simulink model "controller_sim"  (R2022a)
settings: Solver=ode1  StartTime=0.0  StopTime=10.0  FixedStep=0.010  RelTol=1e-5  AbsTol=1e-5
undefined symbols (not defined in the file or in its folder): c_d, c_dn, c_downbound, c_i, c_n, c_p, c_upbound, T0, T1, Td, Tg, Ti, Ts, Tsp, Tsp_delay, Tt
libraries: slpidlib x1
(part 2 of 3)

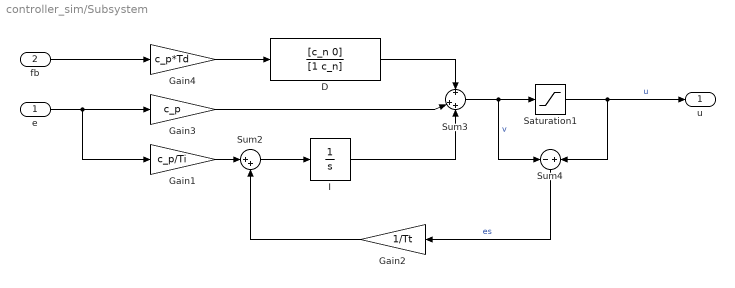
== system controller_sim/Subsystem ==
  e : Inport
  fb : Inport  Port=2
  D : TransferFcn  Numerator=[c_n 0]  Denominator=[1 c_n]
  Gain1 : Gain  Gain=c_p/Ti
  Gain2 : Gain  Gain=1/Tt
  Gain3 : Gain  Gain=c_p
  Gain4 : Gain  Gain=c_p*Td
  I : TransferFcn  Denominator=[1 0]
  Saturation1 : Saturate  UpperLimit=c_upbound  LowerLimit=c_downbound
  Sum2 : Sum  Inputs=|++
  Sum3 : Sum  Inputs=+|++
  Sum4 : Sum  Inputs=-|+
  u : Outport
  wires:
  D/1 -> Sum3/1
  e/1 -> Gain1/1, Gain3/1
  Sum2/1 -> I/1
  Gain4/1 -> D/1
  I/1 -> Sum3/3
  Gain3/1 -> Sum3/2
  Gain1/1 -> Sum2/1
  Saturation1/1 -> u/1, Sum4/2  "u"
  fb/1 -> Gain4/1
  Sum3/1 -> Sum4/1, Saturation1/1  "v"
  Gain2/1 -> Sum2/2
  Sum4/1 -> Gain2/1  "es"

== system controller_sim/Subsystem1 ==
  e : Inport
  fb : Inport  Port=2
  D : TransferFcn  Numerator=[c_n 0]  Denominator=[1 c_n]
  Gain1 : Gain  Gain=c_p/Ti
  Gain2 : Gain  Gain=1/Tt
  Gain3 : Gain  Gain=c_p
  Gain4 : Gain  Gain=c_p*Td
  I : TransferFcn  Denominator=[1 0]
  Saturation1 : Saturate  UpperLimit=c_upbound  LowerLimit=c_downbound
  Sum2 : Sum  Inputs=|++
  Sum3 : Sum  Inputs=+|++
  Sum4 : Sum  Inputs=-|+
  u : Outport
  wires:
  D/1 -> Sum3/1
  e/1 -> Gain1/1, Gain3/1
  Sum2/1 -> I/1
  Gain4/1 -> D/1
  I/1 -> Sum3/3
  Gain3/1 -> Sum3/2
  Gain1/1 -> Sum2/1
  Saturation1/1 -> u/1, Sum4/2  "u"
  fb/1 -> Gain4/1
  Sum3/1 -> Sum4/1, Saturation1/1  "v"
  Gain2/1 -> Sum2/2
  Sum4/1 -> Gain2/1  "es"

== system controller_sim/Subsystem10 ==
  e : Inport
  fb : Inport  Port=2
  D : TransferFcn  Numerator=[c_n]  Denominator=[1 c_n]
  Gain1 : Gain  Gain=c_p/Ti
  Gain2 : Gain  Gain=1/Tt
  Gain3 : Gain  Gain=c_p
  Gain4 : Gain  Gain=c_p*Td
  I : TransferFcn  Denominator=[1 0]
  Saturation1 : Saturate  UpperLimit=c_upbound  LowerLimit=c_downbound
  Sum2 : Sum  Inputs=|++
  Sum3 : Sum  Inputs=+|++
  Sum4 : Sum  Inputs=-|+
  u : Outport
  wires:
  D/1 -> Sum3/1
  e/1 -> Gain1/1, Gain3/1
  Sum2/1 -> I/1
  Gain4/1 -> D/1
  I/1 -> Sum3/3
  Gain3/1 -> Sum3/2
  Gain1/1 -> Sum2/1
  Saturation1/1 -> u/1, Sum4/2  "u"
  fb/1 -> Gain4/1
  Sum3/1 -> Sum4/1, Saturation1/1  "v"
  Gain2/1 -> Sum2/2
  Sum4/1 -> Gain2/1  "es"

== system controller_sim/Subsystem11 ==
  e : Inport
  fb : Inport  Port=2
  D : TransferFcn  Numerator=[c_n]  Denominator=[1 c_n]
  Gain1 : Gain  Gain=c_p/Ti
  Gain2 : Gain  Gain=1/Tt
  Gain3 : Gain  Gain=c_p
  Gain4 : Gain  Gain=c_p*Td
  I : TransferFcn  Denominator=[1 0]
  Saturation1 : Saturate  UpperLimit=c_upbound  LowerLimit=c_downbound
  Sum2 : Sum  Inputs=|++
  Sum3 : Sum  Inputs=+|++
  Sum4 : Sum  Inputs=-|+
  u : Outport
  wires:
  D/1 -> Sum3/1
  e/1 -> Gain1/1, Gain3/1
  Sum2/1 -> I/1
  Gain4/1 -> D/1
  I/1 -> Sum3/3
  Gain3/1 -> Sum3/2
  Gain1/1 -> Sum2/1
  Saturation1/1 -> u/1, Sum4/2  "u"
  fb/1 -> Gain4/1
  Sum3/1 -> Sum4/1, Saturation1/1  "v"
  Gain2/1 -> Sum2/2
  Sum4/1 -> Gain2/1  "es"

== system controller_sim/Subsystem12 ==
  e : Inport
  fb : Inport  Port=2
  D : TransferFcn  Numerator=[c_n]  Denominator=[1 c_n]
  Gain1 : Gain  Gain=c_p/Ti
  Gain2 : Gain  Gain=1/Tt
  Gain3 : Gain  Gain=c_p
  Gain4 : Gain  Gain=c_p*Td
  I : TransferFcn  Denominator=[1 0]
  Saturation1 : Saturate  UpperLimit=c_upbound  LowerLimit=c_downbound
  Sum2 : Sum  Inputs=|++
  Sum3 : Sum  Inputs=+|++
  Sum4 : Sum  Inputs=-|+
  u : Outport
  wires:
  D/1 -> Sum3/1
  e/1 -> Gain1/1, Gain3/1
  Sum2/1 -> I/1
  Gain4/1 -> D/1
  I/1 -> Sum3/3
  Gain3/1 -> Sum3/2
  Gain1/1 -> Sum2/1
  Saturation1/1 -> u/1, Sum4/2  "u"
  fb/1 -> Gain4/1
  Sum3/1 -> Sum4/1, Saturation1/1  "v"
  Gain2/1 -> Sum2/2
  Sum4/1 -> Gain2/1  "es"

== system controller_sim/Subsystem13 ==
  e : Inport
  fb : Inport  Port=2
  D : TransferFcn  Numerator=[c_n 0]  Denominator=[1 c_n]
  Gain1 : Gain  Gain=c_p/Ti
  Gain2 : Gain  Gain=1/Tt
  Gain3 : Gain  Gain=c_p
  Gain4 : Gain  Gain=c_p*Td
  I : TransferFcn  Denominator=[1 0]
  Saturation1 : Saturate  UpperLimit=c_upbound  LowerLimit=c_downbound
  Sum2 : Sum  Inputs=|++
  Sum3 : Sum  Inputs=+|++
  Sum4 : Sum  Inputs=-|+
  u : Outport
  wires:
  D/1 -> Sum3/1
  Sum2/1 -> I/1
  Gain4/1 -> D/1
  I/1 -> Sum3/3
  Gain3/1 -> Sum3/2
  Gain1/1 -> Sum2/1
  Saturation1/1 -> u/1, Sum4/2  "u"
  e/1 -> Gain4/1, Gain1/1, Gain3/1
  Sum3/1 -> Sum4/1, Saturation1/1  "v"
  Gain2/1 -> Sum2/2
  Sum4/1 -> Gain2/1  "es"

== system controller_sim/Subsystem14 ==
  e : Inport
  fb : Inport  Port=2
  D : TransferFcn  Numerator=[c_n 0]  Denominator=[1 c_n]
  Gain1 : Gain  Gain=c_p/Ti
  Gain2 : Gain  Gain=1/Tt
  Gain3 : Gain  Gain=c_p
  Gain4 : Gain  Gain=c_p*Td
  I : TransferFcn  Denominator=[1 0]
  Saturation1 : Saturate  UpperLimit=c_upbound  LowerLimit=c_downbound
  Sum2 : Sum  Inputs=|++
  Sum3 : Sum  Inputs=+|++
  Sum4 : Sum  Inputs=-|+
  u : Outport
  wires:
  D/1 -> Sum3/1
  Sum2/1 -> I/1
  Gain4/1 -> D/1
  I/1 -> Sum3/3
  Gain3/1 -> Sum3/2
  Gain1/1 -> Sum2/1
  Saturation1/1 -> u/1, Sum4/2  "u"
  e/1 -> Gain4/1, Gain1/1, Gain3/1
  Sum3/1 -> Sum4/1, Saturation1/1  "v"
  Gain2/1 -> Sum2/2
  Sum4/1 -> Gain2/1  "es"

== system controller_sim/Subsystem15 ==
  e : Inport
  fb : Inport  Port=2
  D : TransferFcn  Numerator=[c_n 0]  Denominator=[1 c_n]
  Gain1 : Gain  Gain=c_p/Ti
  Gain2 : Gain  Gain=1/Tt
  Gain3 : Gain  Gain=c_p
  Gain4 : Gain  Gain=c_p*Td
  I : TransferFcn  Denominator=[1 0]
  Saturation1 : Saturate  UpperLimit=c_upbound  LowerLimit=c_downbound
  Sum2 : Sum  Inputs=|++
  Sum3 : Sum  Inputs=+|++
  Sum4 : Sum  Inputs=-|+
  u : Outport
  wires:
  Sum4/1 -> Gain2/1  "es"
  Gain2/1 -> Sum2/2
  Sum3/1 -> Saturation1/1, Sum4/1  "v"
  e/1 -> Gain3/1, Gain1/1, Gain4/1
  Saturation1/1 -> Sum4/2, u/1  "u"
  Gain1/1 -> Sum2/1
  Gain3/1 -> Sum3/2
  I/1 -> Sum3/3
  Gain4/1 -> D/1
  Sum2/1 -> I/1
  D/1 -> Sum3/1

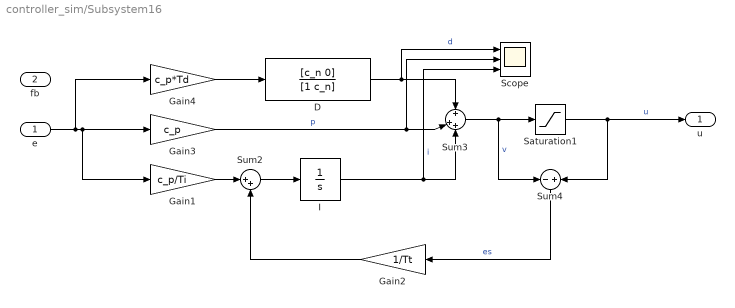
== system controller_sim/Subsystem16 ==
  e : Inport
  fb : Inport  Port=2
  D : TransferFcn  Numerator=[c_n 0]  Denominator=[1 c_n]
  Gain1 : Gain  Gain=c_p/Ti
  Gain2 : Gain  Gain=1/Tt
  Gain3 : Gain  Gain=c_p
  Gain4 : Gain  Gain=c_p*Td
  I : TransferFcn  Denominator=[1 0]
  Saturation1 : Saturate  UpperLimit=c_upbound  LowerLimit=c_downbound
  Scope : Scope  NumInputPorts=3
  Sum2 : Sum  Inputs=|++
  Sum3 : Sum  Inputs=+|++
  Sum4 : Sum  Inputs=-|+
  u : Outport
  wires:
  D/1 -> Scope/1, Sum3/1  "d"
  Sum2/1 -> I/1
  Gain4/1 -> D/1
  I/1 -> Scope/3, Sum3/3  "i"
  Gain3/1 -> Scope/2, Sum3/2  "p"
  Gain1/1 -> Sum2/1
  Saturation1/1 -> u/1, Sum4/2  "u"
  e/1 -> Gain4/1, Gain1/1, Gain3/1
  Sum3/1 -> Sum4/1, Saturation1/1  "v"
  Gain2/1 -> Sum2/2
  Sum4/1 -> Gain2/1  "es"

== system controller_sim/Subsystem17 ==
  e : Inport
  fb : Inport  Port=2
  D : TransferFcn  Numerator=[c_n 0]  Denominator=[1 c_n]
  Gain1 : Gain  Gain=c_p/Ti
  Gain2 : Gain  Gain=1/Tt
  Gain3 : Gain  Gain=c_p
  Gain4 : Gain  Gain=c_p*Td
  I : TransferFcn  Denominator=[1 0]
  Saturation1 : Saturate  UpperLimit=c_upbound  LowerLimit=c_downbound
  Sum2 : Sum  Inputs=|++
  Sum3 : Sum  Inputs=+|++
  Sum4 : Sum  Inputs=-|+
  u : Outport
  wires:
  Sum4/1 -> Gain2/1  "es"
  Gain2/1 -> Sum2/2
  Sum3/1 -> Saturation1/1, Sum4/1  "v"
  e/1 -> Gain3/1, Gain1/1, Gain4/1
  Saturation1/1 -> Sum4/2, u/1  "u"
  Gain1/1 -> Sum2/1
  Gain3/1 -> Sum3/2
  I/1 -> Sum3/3
  Gain4/1 -> D/1
  Sum2/1 -> I/1
  D/1 -> Sum3/1

== system controller_sim/Subsystem18 ==
  e : Inport
  fb : Inport  Port=2
  D : TransferFcn  Numerator=[c_n 0]  Denominator=[1 c_n]
  Gain1 : Gain  Gain=c_p/Ti
  Gain2 : Gain  Gain=1/Tt
  Gain3 : Gain  Gain=c_p
  Gain4 : Gain  Gain=c_p*Td
  I : TransferFcn  Denominator=[1 0]
  Saturation1 : Saturate  UpperLimit=c_upbound  LowerLimit=c_downbound
  Sum2 : Sum  Inputs=|++
  Sum3 : Sum  Inputs=+|++
  Sum4 : Sum  Inputs=-|+
  u : Outport
  wires:
  D/1 -> Sum3/1
  Sum2/1 -> I/1
  Gain4/1 -> D/1
  I/1 -> Sum3/3
  Gain3/1 -> Sum3/2
  Gain1/1 -> Sum2/1
  Saturation1/1 -> u/1, Sum4/2  "u"
  e/1 -> Gain4/1, Gain1/1, Gain3/1
  Sum3/1 -> Sum4/1, Saturation1/1  "v"
  Gain2/1 -> Sum2/2
  Sum4/1 -> Gain2/1  "es"

== system controller_sim/Subsystem19 ==
  e : Inport
  fb : Inport  Port=2
  D : TransferFcn  Numerator=[c_n 0]  Denominator=[1 c_n]
  Gain1 : Gain  Gain=c_p/Ti
  Gain2 : Gain  Gain=1/Tt
  Gain3 : Gain  Gain=c_p
  Gain4 : Gain  Gain=c_p*Td
  I : TransferFcn  Denominator=[1 0]
  Saturation1 : Saturate  UpperLimit=c_upbound  LowerLimit=c_downbound
  Sum2 : Sum  Inputs=|++
  Sum3 : Sum  Inputs=+|++
  Sum4 : Sum  Inputs=-|+
  u : Outport
  wires:
  Sum4/1 -> Gain2/1  "es"
  Gain2/1 -> Sum2/2
  Sum3/1 -> Saturation1/1, Sum4/1  "v"
  e/1 -> Gain3/1, Gain1/1, Gain4/1
  Saturation1/1 -> Sum4/2, u/1  "u"
  Gain1/1 -> Sum2/1
  Gain3/1 -> Sum3/2
  I/1 -> Sum3/3
  Gain4/1 -> D/1
  Sum2/1 -> I/1
  D/1 -> Sum3/1

== system controller_sim/Subsystem2 ==
  e : Inport
  fb : Inport  Port=2
  D : TransferFcn  Numerator=[c_n 0]  Denominator=[1 c_n]
  Gain1 : Gain  Gain=c_p/Ti
  Gain2 : Gain  Gain=1/Tt
  Gain3 : Gain  Gain=c_p
  Gain4 : Gain  Gain=c_p*Td
  I : TransferFcn  Denominator=[1 0]
  Saturation1 : Saturate  UpperLimit=c_upbound  LowerLimit=c_downbound
  Sum2 : Sum  Inputs=|++
  Sum3 : Sum  Inputs=+|++
  Sum4 : Sum  Inputs=-|+
  u : Outport
  wires:
  Sum4/1 -> Gain2/1  "es"
  Gain2/1 -> Sum2/2
  Sum3/1 -> Saturation1/1, Sum4/1  "v"
  fb/1 -> Gain4/1
  Saturation1/1 -> Sum4/2, u/1  "u"
  Gain1/1 -> Sum2/1
  Gain3/1 -> Sum3/2
  I/1 -> Sum3/3
  Gain4/1 -> D/1
  Sum2/1 -> I/1
  e/1 -> Gain3/1, Gain1/1
  D/1 -> Sum3/1

== system controller_sim/Subsystem22 ==
  e : Inport
  fb : Inport  Port=2
  D : TransferFcn  Numerator=[c_n 0]  Denominator=[1 c_n]
  Gain1 : Gain  Gain=c_p/Ti
  Gain2 : Gain  Gain=1/Tt
  Gain3 : Gain  Gain=c_p
  Gain4 : Gain  Gain=c_p*Td
  I : TransferFcn  Denominator=[1 0]
  Saturation1 : Saturate  UpperLimit=c_upbound  LowerLimit=c_downbound
  Sum2 : Sum  Inputs=|++
  Sum3 : Sum  Inputs=+|++
  Sum4 : Sum  Inputs=-|+
  u : Outport
  wires:
  Sum4/1 -> Gain2/1  "es"
  Gain2/1 -> Sum2/2
  Sum3/1 -> Saturation1/1, Sum4/1  "v"
  e/1 -> Gain3/1, Gain1/1, Gain4/1
  Saturation1/1 -> Sum4/2, u/1  "u"
  Gain1/1 -> Sum2/1
  Gain3/1 -> Sum3/2
  I/1 -> Sum3/3
  Gain4/1 -> D/1
  Sum2/1 -> I/1
  D/1 -> Sum3/1

== system controller_sim/Subsystem3 ==
  e : Inport
  fb : Inport  Port=2
  D : TransferFcn  Numerator=[c_n 0]  Denominator=[1 c_n]
  Gain1 : Gain  Gain=c_p/Ti
  Gain2 : Gain  Gain=1/Tt
  Gain3 : Gain  Gain=c_p
  Gain4 : Gain  Gain=c_p*Td
  I : TransferFcn  Denominator=[1 0]
  Saturation1 : Saturate  UpperLimit=c_upbound  LowerLimit=c_downbound
  Sum2 : Sum  Inputs=|++
  Sum3 : Sum  Inputs=+|++
  Sum4 : Sum  Inputs=-|+
  u : Outport
  wires:
  D/1 -> Sum3/1
  e/1 -> Gain1/1, Gain3/1
  Sum2/1 -> I/1
  Gain4/1 -> D/1
  I/1 -> Sum3/3
  Gain3/1 -> Sum3/2
  Gain1/1 -> Sum2/1
  Saturation1/1 -> u/1, Sum4/2  "u"
  fb/1 -> Gain4/1
  Sum3/1 -> Sum4/1, Saturation1/1  "v"
  Gain2/1 -> Sum2/2
  Sum4/1 -> Gain2/1  "es"

== system controller_sim/Subsystem4 ==
  e : Inport
  fb : Inport  Port=2
  D : TransferFcn  Numerator=[c_n]  Denominator=[1 c_n]
  Gain1 : Gain  Gain=c_p/Ti
  Gain2 : Gain  Gain=1/Tt
  Gain3 : Gain  Gain=c_p
  Gain4 : Gain  Gain=c_p*Td
  I : TransferFcn  Denominator=[1 0]
  Saturation1 : Saturate  UpperLimit=c_upbound  LowerLimit=c_downbound
  Sum2 : Sum  Inputs=|++
  Sum3 : Sum  Inputs=+|++
  Sum4 : Sum  Inputs=-|+
  u : Outport
  wires:
  D/1 -> Sum3/1
  e/1 -> Gain1/1, Gain3/1
  Sum2/1 -> I/1
  Gain4/1 -> D/1
  Gain3/1 -> Sum3/2
  Gain1/1 -> Sum2/1
  Saturation1/1 -> Sum3/3, Sum4/2  "u"
  fb/1 -> Gain4/1
  I/1 -> Saturation1/1, Sum4/1  "v"
  Gain2/1 -> Sum2/2
  Sum4/1 -> Gain2/1  "es"
  Sum3/1 -> u/1  "v"

== system controller_sim/Subsystem5 ==
  e : Inport
  fb : Inport  Port=2
  D : TransferFcn  Numerator=[c_n]  Denominator=[1 c_n]
  Gain1 : Gain  Gain=c_p/Ti
  Gain2 : Gain  Gain=1/Tt
  Gain3 : Gain  Gain=c_p
  Gain4 : Gain  Gain=c_p*Td
  I : TransferFcn  Denominator=[1 0]
  Saturation1 : Saturate  UpperLimit=c_upbound  LowerLimit=c_downbound
  Sum2 : Sum  Inputs=|++
  Sum3 : Sum  Inputs=+|++
  Sum4 : Sum  Inputs=-|+
  u : Outport
  wires:
  Sum4/1 -> Gain2/1  "es"
  Gain2/1 -> Sum2/2
  Sum3/1 -> Saturation1/1, Sum4/1  "v"
  fb/1 -> Gain4/1
  Saturation1/1 -> Sum4/2, u/1  "u"
  Gain1/1 -> Sum2/1
  Gain3/1 -> Sum3/2
  I/1 -> Sum3/3
  Gain4/1 -> D/1
  Sum2/1 -> I/1
  e/1 -> Gain3/1, Gain1/1
  D/1 -> Sum3/1

== system controller_sim/Subsystem6 ==
  e : Inport
  fb : Inport  Port=2
  D : TransferFcn  Numerator=[c_n]  Denominator=[1 c_n]
  Gain1 : Gain  Gain=c_p/Ti
  Gain2 : Gain  Gain=1/Tt
  Gain3 : Gain  Gain=c_p
  Gain4 : Gain  Gain=c_p*Td
  I : TransferFcn  Denominator=[1 0]
  Saturation1 : Saturate  UpperLimit=c_upbound  LowerLimit=c_downbound
  Sum2 : Sum  Inputs=|++
  Sum3 : Sum  Inputs=+|++
  Sum4 : Sum  Inputs=-|+
  u : Outport
  wires:
  Sum4/1 -> Gain2/1  "es"
  Gain2/1 -> Sum2/2
  Sum3/1 -> Saturation1/1, Sum4/1  "v"
  fb/1 -> Gain4/1
  Saturation1/1 -> Sum4/2, u/1  "u"
  Gain1/1 -> Sum2/1
  Gain3/1 -> Sum3/2
  I/1 -> Sum3/3
  Gain4/1 -> D/1
  Sum2/1 -> I/1
  e/1 -> Gain3/1, Gain1/1
  D/1 -> Sum3/1

== system controller_sim/Subsystem7 ==
  e : Inport
  fb : Inport  Port=2
  D : TransferFcn  Numerator=[c_n]  Denominator=[1 c_n]
  Gain1 : Gain  Gain=c_p/Ti
  Gain2 : Gain  Gain=1/Tt
  Gain3 : Gain  Gain=c_p
  Gain4 : Gain  Gain=c_p*Td
  I : TransferFcn  Denominator=[1 0]
  Saturation1 : Saturate  UpperLimit=c_upbound  LowerLimit=c_downbound
  Sum2 : Sum  Inputs=|++
  Sum3 : Sum  Inputs=+|++
  Sum4 : Sum  Inputs=-|+
  u : Outport
  wires:
  Sum4/1 -> Gain2/1  "es"
  Gain2/1 -> Sum2/2
  Sum3/1 -> Saturation1/1, Sum4/1  "v"
  fb/1 -> Gain4/1
  Saturation1/1 -> Sum4/2, u/1  "u"
  Gain1/1 -> Sum2/1
  Gain3/1 -> Sum3/2
  I/1 -> Sum3/3
  Gain4/1 -> D/1
  Sum2/1 -> I/1
  e/1 -> Gain3/1, Gain1/1
  D/1 -> Sum3/1

== system controller_sim/Subsystem8 ==
  e : Inport
  fb : Inport  Port=2
  D : TransferFcn  Numerator=[c_n]  Denominator=[1 c_n]
  Gain1 : Gain  Gain=c_p/Ti
  Gain2 : Gain  Gain=1/Tt
  Gain3 : Gain  Gain=c_p
  Gain4 : Gain  Gain=c_p*Td
  I : TransferFcn  Denominator=[1 0]
  Saturation1 : Saturate  UpperLimit=c_upbound  LowerLimit=c_downbound
  Sum2 : Sum  Inputs=|++
  Sum3 : Sum  Inputs=+|++
  Sum4 : Sum  Inputs=-|+
  u : Outport
  wires:
  D/1 -> Sum3/1
  e/1 -> Gain1/1, Gain3/1
  Sum2/1 -> I/1
  Gain4/1 -> D/1
  I/1 -> Sum3/3
  Gain3/1 -> Sum3/2
  Gain1/1 -> Sum2/1
  Saturation1/1 -> u/1, Sum4/2  "u"
  fb/1 -> Gain4/1
  Sum3/1 -> Sum4/1, Saturation1/1  "v"
  Gain2/1 -> Sum2/2
  Sum4/1 -> Gain2/1  "es"

== system controller_sim/Subsystem9 ==
  e : Inport
  fb : Inport  Port=2
  D : TransferFcn  Numerator=[c_n]  Denominator=[1 c_n]
  Gain1 : Gain  Gain=c_p/Ti
  Gain2 : Gain  Gain=1/Tt
  Gain3 : Gain  Gain=c_p
  Gain4 : Gain  Gain=c_p*Td
  I : TransferFcn  Denominator=[1 0]
  Saturation1 : Saturate  UpperLimit=c_upbound  LowerLimit=c_downbound
  Sum2 : Sum  Inputs=|++
  Sum3 : Sum  Inputs=+|++
  Sum4 : Sum  Inputs=-|+
  u : Outport
  wires:
  Sum4/1 -> Gain2/1  "es"
  Gain2/1 -> Sum2/2
  Sum3/1 -> Saturation1/1, Sum4/1  "v"
  fb/1 -> Gain4/1
  Saturation1/1 -> Sum4/2, u/1  "u"
  Gain1/1 -> Sum2/1
  Gain3/1 -> Sum3/2
  I/1 -> Sum3/3
  Gain4/1 -> D/1
  Sum2/1 -> I/1
  e/1 -> Gain3/1, Gain1/1
  D/1 -> Sum3/1

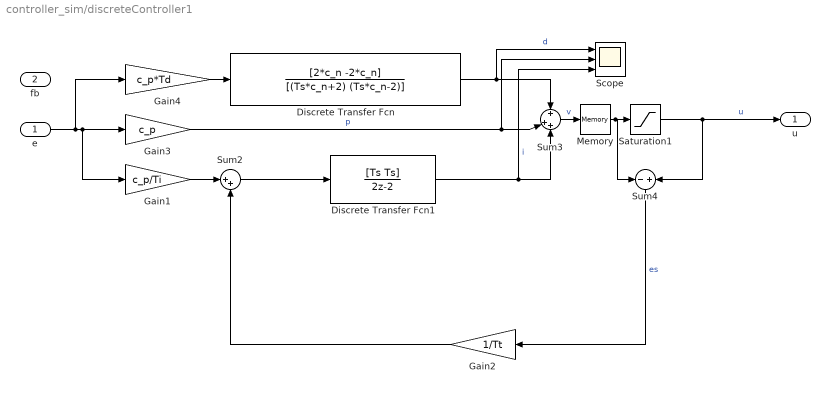
== system controller_sim/discreteController1 ==
  e : Inport
  fb : Inport  Port=2
  Discrete Transfer Fcn : DiscreteTransferFcn  Numerator=[2*c_n -2*c_n]  Denominator=[(Ts*c_n+2) (Ts*c_n-2)]
  Discrete Transfer Fcn1 : DiscreteTransferFcn  Numerator=[Ts Ts]  Denominator=[2 -2]
  Gain1 : Gain  Gain=c_p/Ti
  Gain2 : Gain  Gain=1/Tt
  Gain3 : Gain  Gain=c_p
  Gain4 : Gain  Gain=c_p*Td
  Memory : Memory  InheritSampleTime=on
  Saturation1 : Saturate  UpperLimit=c_upbound  LowerLimit=c_downbound
  Scope : Scope  NumInputPorts=3
  Sum2 : Sum  Inputs=|++
  Sum3 : Sum  Inputs=+|++
  Sum4 : Sum  Inputs=-|+
  u : Outport
  wires:
  Discrete Transfer Fcn/1 -> Scope/1, Sum3/1  "d"
  Sum2/1 -> Discrete Transfer Fcn1/1
  Gain4/1 -> Discrete Transfer Fcn/1
  Discrete Transfer Fcn1/1 -> Scope/3, Sum3/3  "i"
  Gain3/1 -> Scope/2, Sum3/2  "p"
  Gain1/1 -> Sum2/1
  Saturation1/1 -> u/1, Sum4/2  "u"
  e/1 -> Gain4/1, Gain1/1, Gain3/1
  Sum3/1 -> Memory/1  "v"
  Gain2/1 -> Sum2/2
  Sum4/1 -> Gain2/1  "es"
  Memory/1 -> Sum4/1, Saturation1/1

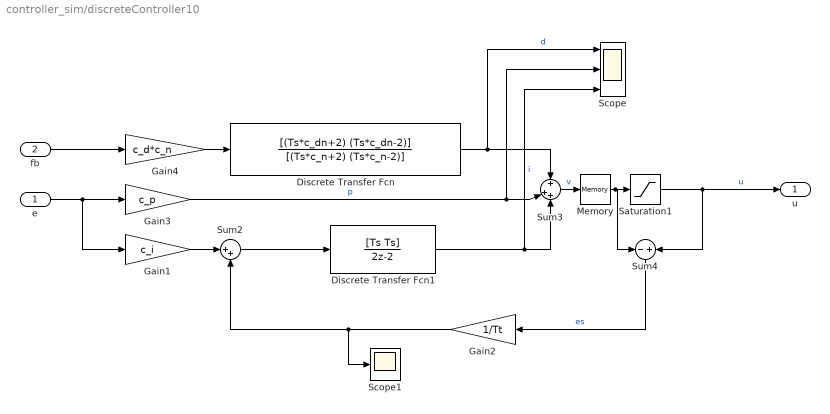
== system controller_sim/discreteController10 ==
  e : Inport
  fb : Inport  Port=2
  Discrete Transfer Fcn : DiscreteTransferFcn  Numerator=[(Ts*c_dn+2) (Ts*c_dn-2)]  Denominator=[(Ts*c_n+2) (Ts*c_n-2)]
  Discrete Transfer Fcn1 : DiscreteTransferFcn  Numerator=[Ts Ts]  Denominator=[2 -2]
  Gain1 : Gain  Gain=c_i
  Gain2 : Gain  Gain=1/Tt
  Gain3 : Gain  Gain=c_p
  Gain4 : Gain  Gain=c_d*c_n
  Memory : Memory  InheritSampleTime=on
  Saturation1 : Saturate  UpperLimit=c_upbound  LowerLimit=c_downbound
  Scope : Scope  NumInputPorts=3
  Scope1 : Scope
  Sum2 : Sum  Inputs=|++
  Sum3 : Sum  Inputs=+|++
  Sum4 : Sum  Inputs=-|+
  u : Outport
  wires:
  Memory/1 -> Saturation1/1, Sum4/1
  Sum4/1 -> Gain2/1  "es"
  Gain2/1 -> Scope1/1, Sum2/2
  Sum3/1 -> Memory/1  "v"
  e/1 -> Gain3/1, Gain1/1
  Saturation1/1 -> Sum4/2, u/1  "u"
  Gain1/1 -> Sum2/1
  Gain3/1 -> Sum3/2, Scope/2  "p"
  Discrete Transfer Fcn1/1 -> Sum3/3, Scope/3  "i"
  Gain4/1 -> Discrete Transfer Fcn/1
  Sum2/1 -> Discrete Transfer Fcn1/1
  Discrete Transfer Fcn/1 -> Sum3/1, Scope/1  "d"
  fb/1 -> Gain4/1

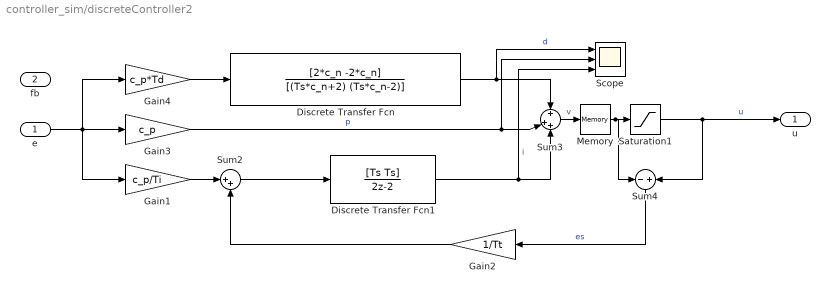
== system controller_sim/discreteController2 ==
  e : Inport
  fb : Inport  Port=2
  Discrete Transfer Fcn : DiscreteTransferFcn  Numerator=[2*c_n -2*c_n]  Denominator=[(Ts*c_n+2) (Ts*c_n-2)]
  Discrete Transfer Fcn1 : DiscreteTransferFcn  Numerator=[Ts Ts]  Denominator=[2 -2]
  Gain1 : Gain  Gain=c_p/Ti
  Gain2 : Gain  Gain=1/Tt
  Gain3 : Gain  Gain=c_p
  Gain4 : Gain  Gain=c_p*Td
  Memory : Memory  InheritSampleTime=on
  Saturation1 : Saturate  UpperLimit=c_upbound  LowerLimit=c_downbound
  Scope : Scope  NumInputPorts=3
  Sum2 : Sum  Inputs=|++
  Sum3 : Sum  Inputs=+|++
  Sum4 : Sum  Inputs=-|+
  u : Outport
  wires:
  Sum4/1 -> Gain2/1  "es"
  Gain2/1 -> Sum2/2
  Sum3/1 -> Memory/1  "v"
  e/1 -> Gain4/1, Gain3/1, Gain1/1
  Saturation1/1 -> Sum4/2, u/1  "u"
  Gain1/1 -> Sum2/1
  Gain3/1 -> Sum3/2, Scope/2  "p"
  Discrete Transfer Fcn1/1 -> Sum3/3, Scope/3  "i"
  Gain4/1 -> Discrete Transfer Fcn/1
  Sum2/1 -> Discrete Transfer Fcn1/1
  Discrete Transfer Fcn/1 -> Sum3/1, Scope/1  "d"
  Memory/1 -> Saturation1/1, Sum4/1

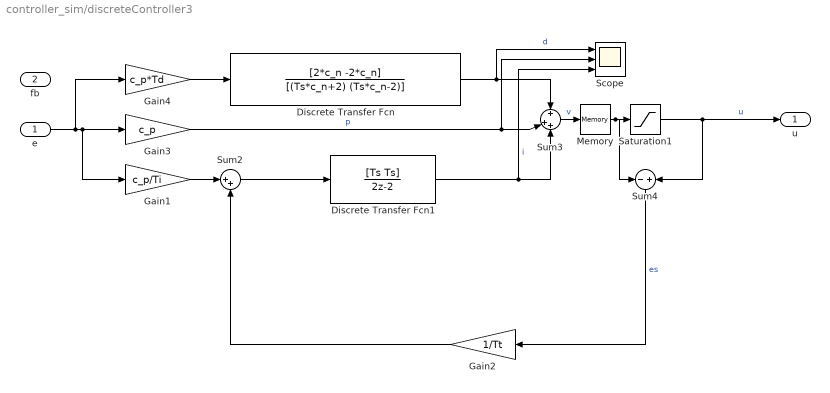
== system controller_sim/discreteController3 ==
  e : Inport
  fb : Inport  Port=2
  Discrete Transfer Fcn : DiscreteTransferFcn  Numerator=[2*c_n -2*c_n]  Denominator=[(Ts*c_n+2) (Ts*c_n-2)]
  Discrete Transfer Fcn1 : DiscreteTransferFcn  Numerator=[Ts Ts]  Denominator=[2 -2]
  Gain1 : Gain  Gain=c_p/Ti
  Gain2 : Gain  Gain=1/Tt
  Gain3 : Gain  Gain=c_p
  Gain4 : Gain  Gain=c_p*Td
  Memory : Memory  InheritSampleTime=on
  Saturation1 : Saturate  UpperLimit=c_upbound  LowerLimit=c_downbound
  Scope : Scope  NumInputPorts=3
  Sum2 : Sum  Inputs=|++
  Sum3 : Sum  Inputs=+|++
  Sum4 : Sum  Inputs=-|+
  u : Outport
  wires:
  Discrete Transfer Fcn/1 -> Scope/1, Sum3/1  "d"
  Sum2/1 -> Discrete Transfer Fcn1/1
  Gain4/1 -> Discrete Transfer Fcn/1
  Discrete Transfer Fcn1/1 -> Scope/3, Sum3/3  "i"
  Gain3/1 -> Scope/2, Sum3/2  "p"
  Gain1/1 -> Sum2/1
  Saturation1/1 -> u/1, Sum4/2  "u"
  e/1 -> Gain4/1, Gain1/1, Gain3/1
  Sum3/1 -> Memory/1  "v"
  Gain2/1 -> Sum2/2
  Sum4/1 -> Gain2/1  "es"
  Memory/1 -> Sum4/1, Saturation1/1

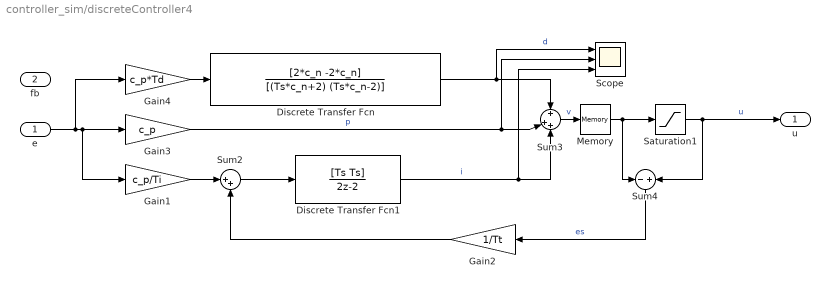
== system controller_sim/discreteController4 ==
  e : Inport
  fb : Inport  Port=2
  Discrete Transfer Fcn : DiscreteTransferFcn  Numerator=[2*c_n -2*c_n]  Denominator=[(Ts*c_n+2) (Ts*c_n-2)]
  Discrete Transfer Fcn1 : DiscreteTransferFcn  Numerator=[Ts Ts]  Denominator=[2 -2]
  Gain1 : Gain  Gain=c_p/Ti
  Gain2 : Gain  Gain=1/Tt
  Gain3 : Gain  Gain=c_p
  Gain4 : Gain  Gain=c_p*Td
  Memory : Memory  InheritSampleTime=on
  Saturation1 : Saturate  UpperLimit=c_upbound  LowerLimit=c_downbound
  Scope : Scope  NumInputPorts=3
  Sum2 : Sum  Inputs=|++
  Sum3 : Sum  Inputs=+|++
  Sum4 : Sum  Inputs=-|+
  u : Outport
  wires:
  Sum4/1 -> Gain2/1  "es"
  Gain2/1 -> Sum2/2
  Sum3/1 -> Memory/1  "v"
  e/1 -> Gain3/1, Gain1/1, Gain4/1
  Saturation1/1 -> Sum4/2, u/1  "u"
  Gain1/1 -> Sum2/1
  Gain3/1 -> Sum3/2, Scope/2  "p"
  Discrete Transfer Fcn1/1 -> Sum3/3, Scope/3  "i"
  Gain4/1 -> Discrete Transfer Fcn/1
  Sum2/1 -> Discrete Transfer Fcn1/1
  Discrete Transfer Fcn/1 -> Sum3/1, Scope/1  "d"
  Memory/1 -> Saturation1/1, Sum4/1

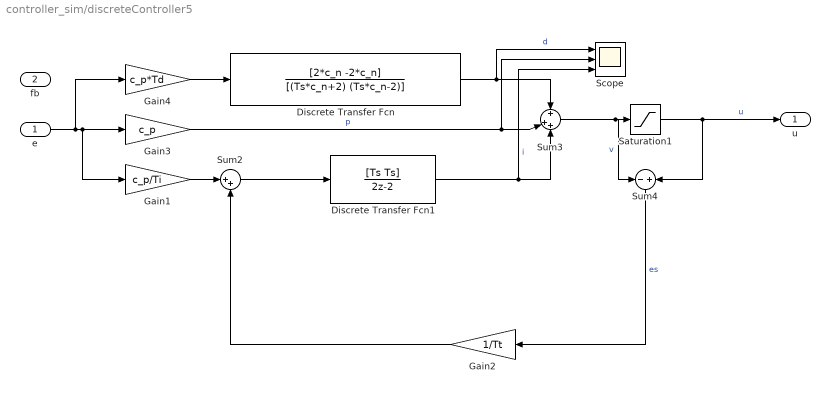
== system controller_sim/discreteController5 ==
  e : Inport
  fb : Inport  Port=2
  Discrete Transfer Fcn : DiscreteTransferFcn  Numerator=[2*c_n -2*c_n]  Denominator=[(Ts*c_n+2) (Ts*c_n-2)]
  Discrete Transfer Fcn1 : DiscreteTransferFcn  Numerator=[Ts Ts]  Denominator=[2 -2]
  Gain1 : Gain  Gain=c_p/Ti
  Gain2 : Gain  Gain=1/Tt
  Gain3 : Gain  Gain=c_p
  Gain4 : Gain  Gain=c_p*Td
  Saturation1 : Saturate  UpperLimit=c_upbound  LowerLimit=c_downbound
  Scope : Scope  NumInputPorts=3
  Sum2 : Sum  Inputs=|++
  Sum3 : Sum  Inputs=+|++
  Sum4 : Sum  Inputs=-|+
  u : Outport
  wires:
  Discrete Transfer Fcn/1 -> Scope/1, Sum3/1  "d"
  Sum2/1 -> Discrete Transfer Fcn1/1
  Gain4/1 -> Discrete Transfer Fcn/1
  Discrete Transfer Fcn1/1 -> Scope/3, Sum3/3  "i"
  Gain3/1 -> Scope/2, Sum3/2  "p"
  Gain1/1 -> Sum2/1
  Saturation1/1 -> u/1, Sum4/2  "u"
  e/1 -> Gain4/1, Gain1/1, Gain3/1
  Sum3/1 -> Sum4/1, Saturation1/1  "v"
  Gain2/1 -> Sum2/2
  Sum4/1 -> Gain2/1  "es"

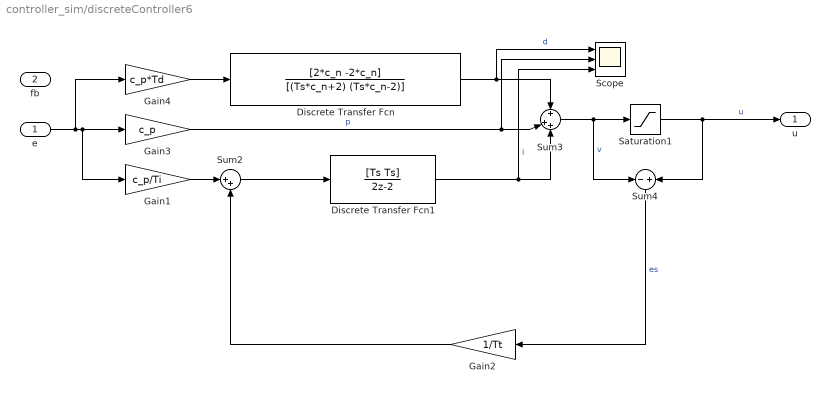
== system controller_sim/discreteController6 ==
  e : Inport
  fb : Inport  Port=2
  Discrete Transfer Fcn : DiscreteTransferFcn  Numerator=[2*c_n -2*c_n]  Denominator=[(Ts*c_n+2) (Ts*c_n-2)]
  Discrete Transfer Fcn1 : DiscreteTransferFcn  Numerator=[Ts Ts]  Denominator=[2 -2]
  Gain1 : Gain  Gain=c_p/Ti
  Gain2 : Gain  Gain=1/Tt
  Gain3 : Gain  Gain=c_p
  Gain4 : Gain  Gain=c_p*Td
  Saturation1 : Saturate  UpperLimit=c_upbound  LowerLimit=c_downbound
  Scope : Scope  NumInputPorts=3
  Sum2 : Sum  Inputs=|++
  Sum3 : Sum  Inputs=+|++
  Sum4 : Sum  Inputs=-|+
  u : Outport
  wires:
  Sum4/1 -> Gain2/1  "es"
  Gain2/1 -> Sum2/2
  Sum3/1 -> Saturation1/1, Sum4/1  "v"
  e/1 -> Gain3/1, Gain1/1, Gain4/1
  Saturation1/1 -> Sum4/2, u/1  "u"
  Gain1/1 -> Sum2/1
  Gain3/1 -> Sum3/2, Scope/2  "p"
  Discrete Transfer Fcn1/1 -> Sum3/3, Scope/3  "i"
  Gain4/1 -> Discrete Transfer Fcn/1
  Sum2/1 -> Discrete Transfer Fcn1/1
  Discrete Transfer Fcn/1 -> Sum3/1, Scope/1  "d"

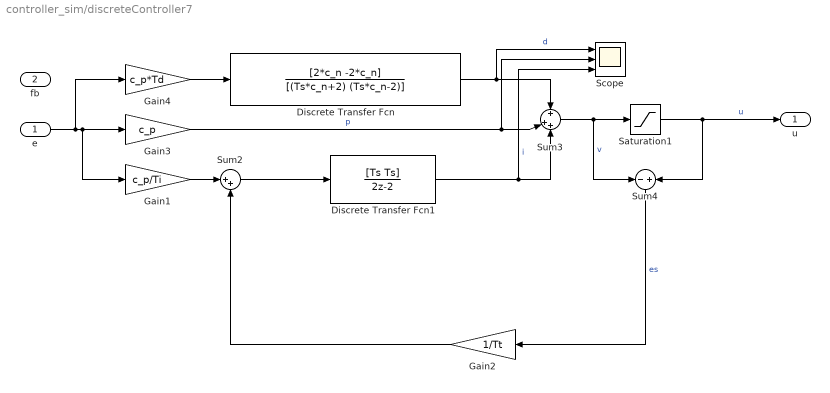
== system controller_sim/discreteController7 ==
  e : Inport
  fb : Inport  Port=2
  Discrete Transfer Fcn : DiscreteTransferFcn  Numerator=[2*c_n -2*c_n]  Denominator=[(Ts*c_n+2) (Ts*c_n-2)]
  Discrete Transfer Fcn1 : DiscreteTransferFcn  Numerator=[Ts Ts]  Denominator=[2 -2]
  Gain1 : Gain  Gain=c_p/Ti
  Gain2 : Gain  Gain=1/Tt
  Gain3 : Gain  Gain=c_p
  Gain4 : Gain  Gain=c_p*Td
  Saturation1 : Saturate  UpperLimit=c_upbound  LowerLimit=c_downbound
  Scope : Scope  NumInputPorts=3
  Sum2 : Sum  Inputs=|++
  Sum3 : Sum  Inputs=+|++
  Sum4 : Sum  Inputs=-|+
  u : Outport
  wires:
  Discrete Transfer Fcn/1 -> Scope/1, Sum3/1  "d"
  Sum2/1 -> Discrete Transfer Fcn1/1
  Gain4/1 -> Discrete Transfer Fcn/1
  Discrete Transfer Fcn1/1 -> Scope/3, Sum3/3  "i"
  Gain3/1 -> Scope/2, Sum3/2  "p"
  Gain1/1 -> Sum2/1
  Saturation1/1 -> u/1, Sum4/2  "u"
  e/1 -> Gain4/1, Gain1/1, Gain3/1
  Sum3/1 -> Sum4/1, Saturation1/1  "v"
  Gain2/1 -> Sum2/2
  Sum4/1 -> Gain2/1  "es"

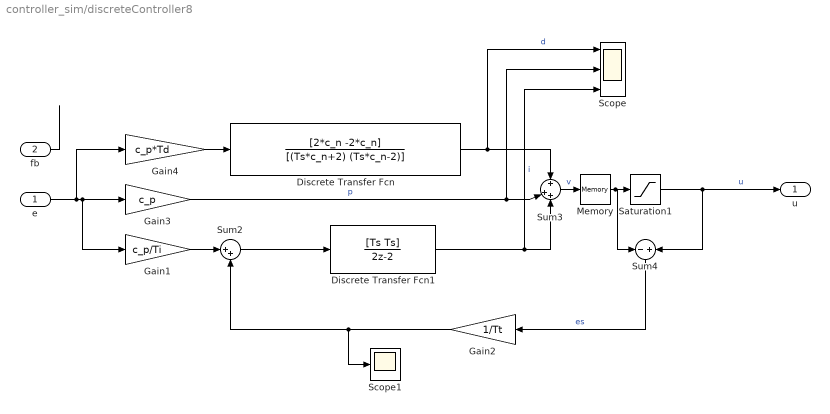
== system controller_sim/discreteController8 ==
  e : Inport
  fb : Inport  Port=2
  Discrete Transfer Fcn : DiscreteTransferFcn  Numerator=[2*c_n -2*c_n]  Denominator=[(Ts*c_n+2) (Ts*c_n-2)]
  Discrete Transfer Fcn1 : DiscreteTransferFcn  Numerator=[Ts Ts]  Denominator=[2 -2]
  Gain1 : Gain  Gain=c_p/Ti
  Gain2 : Gain  Gain=1/Tt
  Gain3 : Gain  Gain=c_p
  Gain4 : Gain  Gain=c_p*Td
  Memory : Memory  InheritSampleTime=on
  Saturation1 : Saturate  UpperLimit=c_upbound  LowerLimit=c_downbound
  Scope : Scope  NumInputPorts=3
  Scope1 : Scope
  Sum2 : Sum  Inputs=|++
  Sum3 : Sum  Inputs=+|++
  Sum4 : Sum  Inputs=-|+
  u : Outport
  wires:
  Memory/1 -> Saturation1/1, Sum4/1
  Sum4/1 -> Gain2/1  "es"
  Gain2/1 -> Scope1/1, Sum2/2
  Sum3/1 -> Memory/1  "v"
  e/1 -> Gain4/1, Gain3/1, Gain1/1
  Saturation1/1 -> Sum4/2, u/1  "u"
  Gain1/1 -> Sum2/1
  Gain3/1 -> Sum3/2, Scope/2  "p"
  Discrete Transfer Fcn1/1 -> Sum3/3, Scope/3  "i"
  Gain4/1 -> Discrete Transfer Fcn/1
  Sum2/1 -> Discrete Transfer Fcn1/1
  Discrete Transfer Fcn/1 -> Sum3/1, Scope/1  "d"
  fb/1 -> ?

== matlab function controller_sim/427wrpm2throttle4 ==
  data: u input; y output
function y = fcn(u)
wrpm = u;
wrpm_430 = [3.50000000000000;4.10000000000000;4.70000000000000;5.30000000000000;5.80000000000000;6.30000000000000;6.80000000000000;7.10000000000000;7.50000000000000;7.80000000000000;8.20000000000000;8.40000000000000;8.70000000000000;8.80000000000000;9;9.10000000000000;9.30000000000000;9.40000000000000;9.50000000000000;9.60000000000000;9.70000000000000];
throttle_430 = [0;0.0500000000000000;0.100000000000000;0.150000000000000;0.200000000000000;0.250000000000000;0.300000000000000;0.350000000000000;0.400000000000000;0.450000000000000;0.500000000000000;0.550000000000000;0.600000000000000;0.650000000000000;0.700000000000000;0.750000000000000;0.800000000000000;0.850000000000000;0.900000000000000;0.950000000000000;1];

y = interp1(  wrpm_430, throttle_430, wrpm, 'linear')*1000;

== matlab function controller_sim/426throttle2wrpm1 ==
  data: u input; y output
function y = fcn(u)
throttle = u/1000.0;
wrpm_430 = [3.60000000000000;4.20000000000000;4.70000000000000;5.20000000000000;5.70000000000000;6.10000000000000;6.50000000000000;6.90000000000000;7.20000000000000;7.50000000000000;7.80000000000000;8.10000000000000;8.30000000000000;8.50000000000000;8.70000000000000;8.90000000000000;9;9.20000000000000;9.30000000000000;9.40000000000000;9.70000000000000];
throttle_430 = [0;0.0500000000000000;0.100000000000000;0.150000000000000;0.200000000000000;0.250000000000000;0.300000000000000;0.350000000000000;0.400000000000000;0.450000000000000;0.500000000000000;0.550000000000000;0.600000000000000;0.650000000000000;0.700000000000000;0.750000000000000;0.800000000000000;0.850000000000000;0.900000000000000;0.950000000000000;1];
y = interp1(throttle_430, wrpm_430, throttle, 'linear');

== matlab function controller_sim/426wrpm2throttle2 ==
  data: u input; y output
function y = fcn(u)
wrpm = u;
wrpm_430 = [3.60000000000000;4.20000000000000;4.70000000000000;5.20000000000000;5.70000000000000;6.10000000000000;6.50000000000000;6.90000000000000;7.20000000000000;7.50000000000000;7.80000000000000;8.10000000000000;8.30000000000000;8.50000000000000;8.70000000000000;8.90000000000000;9;9.20000000000000;9.30000000000000;9.40000000000000;9.70000000000000];
throttle_430 = [0;0.0500000000000000;0.100000000000000;0.150000000000000;0.200000000000000;0.250000000000000;0.300000000000000;0.350000000000000;0.400000000000000;0.450000000000000;0.500000000000000;0.550000000000000;0.600000000000000;0.650000000000000;0.700000000000000;0.750000000000000;0.800000000000000;0.850000000000000;0.900000000000000;0.950000000000000;1];

y = interp1(  wrpm_430, throttle_430, wrpm, 'linear')*1000;

== matlab function controller_sim/426wrpm2throttle3 ==
  data: u input; y output
function y = fcn(u)
wrpm = u;
wrpm_430 = [3.60000000000000;4.20000000000000;4.70000000000000;5.20000000000000;5.70000000000000;6.10000000000000;6.50000000000000;6.90000000000000;7.20000000000000;7.50000000000000;7.80000000000000;8.10000000000000;8.30000000000000;8.50000000000000;8.70000000000000;8.90000000000000;9;9.20000000000000;9.30000000000000;9.40000000000000;9.70000000000000];
throttle_430 = [0;0.0500000000000000;0.100000000000000;0.150000000000000;0.200000000000000;0.250000000000000;0.300000000000000;0.350000000000000;0.400000000000000;0.450000000000000;0.500000000000000;0.550000000000000;0.600000000000000;0.650000000000000;0.700000000000000;0.750000000000000;0.800000000000000;0.850000000000000;0.900000000000000;0.950000000000000;1];

y = interp1(  wrpm_430, throttle_430, wrpm, 'linear')*1000;

== matlab function controller_sim/015throttle2wrpm2 ==
  data: u input; y output
function y = fcn(u)
throttle = u/1000.0;
wrpm_430 = [3.60000000000000;4.70000000000000;5.20000000000000;5.70000000000000;6.20000000000000;6.60000000000000;7;7.30000000000000;7.60000000000000;7.90000000000000;8.10000000000000;8.40000000000000;8.60000000000000;8.80000000000000;8.90000000000000;9;9.20000000000000;9.30000000000000;9.40000000000000;9.50000000000000;9.70000000000000];
throttle_430 = [0;0.0500000000000000;0.100000000000000;0.150000000000000;0.200000000000000;0.250000000000000;0.300000000000000;0.350000000000000;0.400000000000000;0.450000000000000;0.500000000000000;0.550000000000000;0.600000000000000;0.650000000000000;0.700000000000000;0.750000000000000;0.800000000000000;0.850000000000000;0.900000000000000;0.950000000000000;1];
y = interp1(throttle_430, wrpm_430, throttle, 'linear');

== matlab function controller_sim/015wrpm2throttle1 ==
  data: u input; y output
function y = fcn(u)
wrpm = u;
wrpm_430 = [3.60000000000000;4.70000000000000;5.20000000000000;5.70000000000000;6.20000000000000;6.60000000000000;7;7.30000000000000;7.60000000000000;7.90000000000000;8.10000000000000;8.40000000000000;8.60000000000000;8.80000000000000;8.90000000000000;9;9.20000000000000;9.30000000000000;9.40000000000000;9.50000000000000;9.70000000000000];
throttle_430 = [0;0.0500000000000000;0.100000000000000;0.150000000000000;0.200000000000000;0.250000000000000;0.300000000000000;0.350000000000000;0.400000000000000;0.450000000000000;0.500000000000000;0.550000000000000;0.600000000000000;0.650000000000000;0.700000000000000;0.750000000000000;0.800000000000000;0.850000000000000;0.900000000000000;0.950000000000000;1];

y = interp1(  wrpm_430, throttle_430, wrpm, 'linear')*1000;

== matlab function controller_sim/015wrpm2throttle4 ==
  data: u input; y output
function y = fcn(u)
wrpm = u;
wrpm_430 = [3.60000000000000;4.70000000000000;5.20000000000000;5.70000000000000;6.20000000000000;6.60000000000000;7;7.30000000000000;7.60000000000000;7.90000000000000;8.10000000000000;8.40000000000000;8.60000000000000;8.80000000000000;8.90000000000000;9;9.20000000000000;9.30000000000000;9.40000000000000;9.50000000000000;9.70000000000000];
throttle_430 = [0;0.0500000000000000;0.100000000000000;0.150000000000000;0.200000000000000;0.250000000000000;0.300000000000000;0.350000000000000;0.400000000000000;0.450000000000000;0.500000000000000;0.550000000000000;0.600000000000000;0.650000000000000;0.700000000000000;0.750000000000000;0.800000000000000;0.850000000000000;0.900000000000000;0.950000000000000;1];

y = interp1(  wrpm_430, throttle_430, wrpm, 'linear')*1000;

== matlab function controller_sim/431throttle2wrpm ==
  data: u input; y output
function y = fcn(u)
throttle = u/1000.0;
wrpm_431 = [3.6;4.2;4.7;5.2;5.7;6.2;6.5;7;7.3;7.6;7.9;8.2;8.4;8.7;8.9;9;9.2;9.3;9.4;9.5;9.7];
throttle_431 = [0;0.05;0.1;0.15;0.2;0.25;0.3;0.35;0.4;0.45;0.5;0.55;0.6;0.65;0.7;0.75;0.8;0.85;0.9;0.95;1];
y = interp1(throttle_431, wrpm_431, throttle, 'linear');

== matlab function controller_sim/013throttle2wrpm1 ==
  data: u input; y output
function y = fcn(u)
throttle = u/1000.0;
wrpm_430 = [3.50000000000000;4;4.50000000000000;5.10000000000000;5.60000000000000;6.10000000000000;6.50000000000000;7;7.30000000000000;7.80000000000000;8;8.30000000000000;8.50000000000000;8.70000000000000;8.90000000000000;9.10000000000000;9.30000000000000;9.40000000000000;9.50000000000000;9.60000000000000;9.70000000000000];
throttle_430 = [0;0.0500000000000000;0.100000000000000;0.150000000000000;0.200000000000000;0.250000000000000;0.300000000000000;0.350000000000000;0.400000000000000;0.450000000000000;0.500000000000000;0.550000000000000;0.600000000000000;0.650000000000000;0.700000000000000;0.750000000000000;0.800000000000000;0.850000000000000;0.900000000000000;0.950000000000000;1];
y = interp1(throttle_430, wrpm_430, throttle, 'linear');

== matlab function controller_sim/013wrpm2throttle2 ==
  data: u input; y output
function y = fcn(u)
wrpm = u;
wrpm_430 = [3.50000000000000;4;4.50000000000000;5.10000000000000;5.60000000000000;6.10000000000000;6.50000000000000;7;7.30000000000000;7.80000000000000;8;8.30000000000000;8.50000000000000;8.70000000000000;8.90000000000000;9.10000000000000;9.30000000000000;9.40000000000000;9.50000000000000;9.60000000000000;9.70000000000000];
throttle_430 = [0;0.0500000000000000;0.100000000000000;0.150000000000000;0.200000000000000;0.250000000000000;0.300000000000000;0.350000000000000;0.400000000000000;0.450000000000000;0.500000000000000;0.550000000000000;0.600000000000000;0.650000000000000;0.700000000000000;0.750000000000000;0.800000000000000;0.850000000000000;0.900000000000000;0.950000000000000;1];

y = interp1(  wrpm_430, throttle_430, wrpm, 'linear')*1000;

== matlab function controller_sim/013wrpm2throttle3 ==
  data: u input; y output
function y = fcn(u)
wrpm = u;
wrpm_430 = [3.50000000000000;4;4.50000000000000;5.10000000000000;5.60000000000000;6.10000000000000;6.50000000000000;7;7.30000000000000;7.80000000000000;8;8.30000000000000;8.50000000000000;8.70000000000000;8.90000000000000;9.10000000000000;9.30000000000000;9.40000000000000;9.50000000000000;9.60000000000000;9.70000000000000];
throttle_430 = [0;0.0500000000000000;0.100000000000000;0.150000000000000;0.200000000000000;0.250000000000000;0.300000000000000;0.350000000000000;0.400000000000000;0.450000000000000;0.500000000000000;0.550000000000000;0.600000000000000;0.650000000000000;0.700000000000000;0.750000000000000;0.800000000000000;0.850000000000000;0.900000000000000;0.950000000000000;1];

y = interp1(  wrpm_430, throttle_430, wrpm, 'linear')*1000;

== matlab function controller_sim/013throttle2wrpm2 ==
  data: u input; y output
function y = fcn(u)
throttle = u/1000.0;
wrpm_430 = [3.50000000000000;4;4.50000000000000;5.10000000000000;5.60000000000000;6.10000000000000;6.50000000000000;7;7.30000000000000;7.80000000000000;8;8.30000000000000;8.50000000000000;8.70000000000000;8.90000000000000;9.10000000000000;9.30000000000000;9.40000000000000;9.50000000000000;9.60000000000000;9.70000000000000];
throttle_430 = [0;0.0500000000000000;0.100000000000000;0.150000000000000;0.200000000000000;0.250000000000000;0.300000000000000;0.350000000000000;0.400000000000000;0.450000000000000;0.500000000000000;0.550000000000000;0.600000000000000;0.650000000000000;0.700000000000000;0.750000000000000;0.800000000000000;0.850000000000000;0.900000000000000;0.950000000000000;1];
y = interp1(throttle_430, wrpm_430, throttle, 'linear');

== matlab function controller_sim/427wrpm2throttle13 ==
  data: u input; y output
function y = fcn(u)
wrpm = u;
wrpm_430 = [3.50000000000000;4.10000000000000;4.70000000000000;5.30000000000000;5.80000000000000;6.30000000000000;6.80000000000000;7.10000000000000;7.50000000000000;7.80000000000000;8.20000000000000;8.40000000000000;8.70000000000000;8.80000000000000;9;9.10000000000000;9.30000000000000;9.40000000000000;9.50000000000000;9.60000000000000;9.70000000000000];
throttle_430 = [0;0.0500000000000000;0.100000000000000;0.150000000000000;0.200000000000000;0.250000000000000;0.300000000000000;0.350000000000000;0.400000000000000;0.450000000000000;0.500000000000000;0.550000000000000;0.600000000000000;0.650000000000000;0.700000000000000;0.750000000000000;0.800000000000000;0.850000000000000;0.900000000000000;0.950000000000000;1];

y = interp1(  wrpm_430, throttle_430, wrpm, 'linear')*1000;

== matlab function controller_sim/427wrpm2throttle14 ==
  data: u input; y output
function y = fcn(u)
wrpm = u;
wrpm_430 = [3.50000000000000;4.10000000000000;4.70000000000000;5.30000000000000;5.80000000000000;6.30000000000000;6.80000000000000;7.10000000000000;7.50000000000000;7.80000000000000;8.20000000000000;8.40000000000000;8.70000000000000;8.80000000000000;9;9.10000000000000;9.30000000000000;9.40000000000000;9.50000000000000;9.60000000000000;9.70000000000000];
throttle_430 = [0;0.0500000000000000;0.100000000000000;0.150000000000000;0.200000000000000;0.250000000000000;0.300000000000000;0.350000000000000;0.400000000000000;0.450000000000000;0.500000000000000;0.550000000000000;0.600000000000000;0.650000000000000;0.700000000000000;0.750000000000000;0.800000000000000;0.850000000000000;0.900000000000000;0.950000000000000;1];

y = interp1(  wrpm_430, throttle_430, wrpm, 'linear')*1000;

== matlab function controller_sim/015throttle2wrpm1 ==
  data: u input; y output
function y = fcn(u)
throttle = u/1000.0;
wrpm_430 = [3.60000000000000;4.70000000000000;5.20000000000000;5.70000000000000;6.20000000000000;6.60000000000000;7;7.30000000000000;7.60000000000000;7.90000000000000;8.10000000000000;8.40000000000000;8.60000000000000;8.80000000000000;8.90000000000000;9;9.20000000000000;9.30000000000000;9.40000000000000;9.50000000000000;9.70000000000000];
throttle_430 = [0;0.0500000000000000;0.100000000000000;0.150000000000000;0.200000000000000;0.250000000000000;0.300000000000000;0.350000000000000;0.400000000000000;0.450000000000000;0.500000000000000;0.550000000000000;0.600000000000000;0.650000000000000;0.700000000000000;0.750000000000000;0.800000000000000;0.850000000000000;0.900000000000000;0.950000000000000;1];
y = interp1(throttle_430, wrpm_430, throttle, 'linear');

== matlab function controller_sim/427wrpm2throttle15 ==
  data: u input; y output
function y = fcn(u)
wrpm = u;
wrpm_430 = [3.50000000000000;4.10000000000000;4.70000000000000;5.30000000000000;5.80000000000000;6.30000000000000;6.80000000000000;7.10000000000000;7.50000000000000;7.80000000000000;8.20000000000000;8.40000000000000;8.70000000000000;8.80000000000000;9;9.10000000000000;9.30000000000000;9.40000000000000;9.50000000000000;9.60000000000000;9.70000000000000];
throttle_430 = [0;0.0500000000000000;0.100000000000000;0.150000000000000;0.200000000000000;0.250000000000000;0.300000000000000;0.350000000000000;0.400000000000000;0.450000000000000;0.500000000000000;0.550000000000000;0.600000000000000;0.650000000000000;0.700000000000000;0.750000000000000;0.800000000000000;0.850000000000000;0.900000000000000;0.950000000000000;1];

y = interp1(  wrpm_430, throttle_430, wrpm, 'linear')*1000;

== matlab function controller_sim/427wrpm2throttle16 ==
  data: u input; y output
function y = fcn(u)
wrpm = u;
wrpm_430 = [3.50000000000000;4.10000000000000;4.70000000000000;5.30000000000000;5.80000000000000;6.30000000000000;6.80000000000000;7.10000000000000;7.50000000000000;7.80000000000000;8.20000000000000;8.40000000000000;8.70000000000000;8.80000000000000;9;9.10000000000000;9.30000000000000;9.40000000000000;9.50000000000000;9.60000000000000;9.70000000000000];
throttle_430 = [0;0.0500000000000000;0.100000000000000;0.150000000000000;0.200000000000000;0.250000000000000;0.300000000000000;0.350000000000000;0.400000000000000;0.450000000000000;0.500000000000000;0.550000000000000;0.600000000000000;0.650000000000000;0.700000000000000;0.750000000000000;0.800000000000000;0.850000000000000;0.900000000000000;0.950000000000000;1];

y = interp1(  wrpm_430, throttle_430, wrpm, 'linear')*1000;

== matlab function controller_sim/426throttle2wrpm2 ==
  data: u input; y output
function y = fcn(u)
throttle = u/1000.0;
wrpm_430 = [3.60000000000000;4.20000000000000;4.70000000000000;5.20000000000000;5.70000000000000;6.10000000000000;6.50000000000000;6.90000000000000;7.20000000000000;7.50000000000000;7.80000000000000;8.10000000000000;8.30000000000000;8.50000000000000;8.70000000000000;8.90000000000000;9;9.20000000000000;9.30000000000000;9.40000000000000;9.70000000000000];
throttle_430 = [0;0.0500000000000000;0.100000000000000;0.150000000000000;0.200000000000000;0.250000000000000;0.300000000000000;0.350000000000000;0.400000000000000;0.450000000000000;0.500000000000000;0.550000000000000;0.600000000000000;0.650000000000000;0.700000000000000;0.750000000000000;0.800000000000000;0.850000000000000;0.900000000000000;0.950000000000000;1];
y = interp1(throttle_430, wrpm_430, throttle, 'linear');

== matlab function controller_sim/431wrpm2throttle1 ==
  data: u input; y output
function y = fcn(u)
wrpm = u;
wrpm_431 = [3.6;4.2;4.7;5.2;5.7;6.2;6.5;7;7.3;7.6;7.9;8.2;8.4;8.7;8.9;9;9.2;9.3;9.4;9.5;9.7];
throttle_431 = [0;0.05;0.1;0.15;0.2;0.25;0.3;0.35;0.4;0.45;0.5;0.55;0.6;0.65;0.7;0.75;0.8;0.85;0.9;0.95;1];

y = interp1(  wrpm_431, throttle_431, wrpm, 'linear')*1000;

== matlab function controller_sim/427wrpm2throttle2 ==
  data: u input; y output
function y = fcn(u)
wrpm = u;
wrpm_430 = [3.50000000000000;4.10000000000000;4.70000000000000;5.30000000000000;5.80000000000000;6.30000000000000;6.80000000000000;7.10000000000000;7.50000000000000;7.80000000000000;8.20000000000000;8.40000000000000;8.70000000000000;8.80000000000000;9;9.10000000000000;9.30000000000000;9.40000000000000;9.50000000000000;9.60000000000000;9.70000000000000];
throttle_430 = [0;0.0500000000000000;0.100000000000000;0.150000000000000;0.200000000000000;0.250000000000000;0.300000000000000;0.350000000000000;0.400000000000000;0.450000000000000;0.500000000000000;0.550000000000000;0.600000000000000;0.650000000000000;0.700000000000000;0.750000000000000;0.800000000000000;0.850000000000000;0.900000000000000;0.950000000000000;1];

y = interp1(  wrpm_430, throttle_430, wrpm, 'linear')*1000;

== matlab function controller_sim/427wrpm2throttle11 ==
  data: u input; y output
function y = fcn(u)
wrpm = u;
wrpm_430 = [3.50000000000000;4.10000000000000;4.70000000000000;5.30000000000000;5.80000000000000;6.30000000000000;6.80000000000000;7.10000000000000;7.50000000000000;7.80000000000000;8.20000000000000;8.40000000000000;8.70000000000000;8.80000000000000;9;9.10000000000000;9.30000000000000;9.40000000000000;9.50000000000000;9.60000000000000;9.70000000000000];
throttle_430 = [0;0.0500000000000000;0.100000000000000;0.150000000000000;0.200000000000000;0.250000000000000;0.300000000000000;0.350000000000000;0.400000000000000;0.450000000000000;0.500000000000000;0.550000000000000;0.600000000000000;0.650000000000000;0.700000000000000;0.750000000000000;0.800000000000000;0.850000000000000;0.900000000000000;0.950000000000000;1];

y = interp1(  wrpm_430, throttle_430, wrpm, 'linear')*1000;

== matlab function controller_sim/427throttle2wrpm1 ==
  data: u input; y output
function y = fcn(u)
throttle = u/1000.0;
wrpm_430 = [3.50000000000000;4.10000000000000;4.70000000000000;5.30000000000000;5.80000000000000;6.30000000000000;6.80000000000000;7.10000000000000;7.50000000000000;7.80000000000000;8.20000000000000;8.40000000000000;8.70000000000000;8.80000000000000;9;9.10000000000000;9.30000000000000;9.40000000000000;9.50000000000000;9.60000000000000;9.70000000000000];
throttle_430 = [0;0.0500000000000000;0.100000000000000;0.150000000000000;0.200000000000000;0.250000000000000;0.300000000000000;0.350000000000000;0.400000000000000;0.450000000000000;0.500000000000000;0.550000000000000;0.600000000000000;0.650000000000000;0.700000000000000;0.750000000000000;0.800000000000000;0.850000000000000;0.900000000000000;0.950000000000000;1];
y = interp1(throttle_430, wrpm_430, throttle, 'linear');

== matlab function controller_sim/427wrpm2throttle9 ==
  data: u input; y output
function y = fcn(u)
wrpm = u;
wrpm_430 = [3.50000000000000;4.10000000000000;4.70000000000000;5.30000000000000;5.80000000000000;6.30000000000000;6.80000000000000;7.10000000000000;7.50000000000000;7.80000000000000;8.20000000000000;8.40000000000000;8.70000000000000;8.80000000000000;9;9.10000000000000;9.30000000000000;9.40000000000000;9.50000000000000;9.60000000000000;9.70000000000000];
throttle_430 = [0;0.0500000000000000;0.100000000000000;0.150000000000000;0.200000000000000;0.250000000000000;0.300000000000000;0.350000000000000;0.400000000000000;0.450000000000000;0.500000000000000;0.550000000000000;0.600000000000000;0.650000000000000;0.700000000000000;0.750000000000000;0.800000000000000;0.850000000000000;0.900000000000000;0.950000000000000;1];

y = interp1(  wrpm_430, throttle_430, wrpm, 'linear')*1000;

== matlab function controller_sim/427wrpm2throttle10 ==
  data: u input; y output
function y = fcn(u)
wrpm = u;
wrpm_430 = [3.50000000000000;4.10000000000000;4.70000000000000;5.30000000000000;5.80000000000000;6.30000000000000;6.80000000000000;7.10000000000000;7.50000000000000;7.80000000000000;8.20000000000000;8.40000000000000;8.70000000000000;8.80000000000000;9;9.10000000000000;9.30000000000000;9.40000000000000;9.50000000000000;9.60000000000000;9.70000000000000];
throttle_430 = [0;0.0500000000000000;0.100000000000000;0.150000000000000;0.200000000000000;0.250000000000000;0.300000000000000;0.350000000000000;0.400000000000000;0.450000000000000;0.500000000000000;0.550000000000000;0.600000000000000;0.650000000000000;0.700000000000000;0.750000000000000;0.800000000000000;0.850000000000000;0.900000000000000;0.950000000000000;1];

y = interp1(  wrpm_430, throttle_430, wrpm, 'linear')*1000;

== matlab function controller_sim/428throttle2wrpm2 ==
  data: u input; y output
function y = fcn(u)
throttle = u/1000.0;
wrpm_430 = [3.58000000000000;4.30000000000000;4.90000000000000;5.40000000000000;6;6.40000000000000;6.90000000000000;7.20000000000000;7.50000000000000;7.90000000000000;8.20000000000000;8.50000000000000;8.80000000000000;8.90000000000000;9;9.20000000000000;9.30000000000000;9.40000000000000;9.50000000000000;9.60000000000000;9.70000000000000];
throttle_430 = [0;0.0500000000000000;0.100000000000000;0.150000000000000;0.200000000000000;0.250000000000000;0.300000000000000;0.350000000000000;0.400000000000000;0.450000000000000;0.500000000000000;0.550000000000000;0.600000000000000;0.650000000000000;0.700000000000000;0.750000000000000;0.800000000000000;0.850000000000000;0.900000000000000;0.950000000000000;1];
y = interp1(throttle_430, wrpm_430, throttle, 'linear');

== matlab function controller_sim/427wrpm2throttle7 ==
  data: u input; y output
function y = fcn(u)
wrpm = u;
wrpm_430 = [3.50000000000000;4.10000000000000;4.70000000000000;5.30000000000000;5.80000000000000;6.30000000000000;6.80000000000000;7.10000000000000;7.50000000000000;7.80000000000000;8.20000000000000;8.40000000000000;8.70000000000000;8.80000000000000;9;9.10000000000000;9.30000000000000;9.40000000000000;9.50000000000000;9.60000000000000;9.70000000000000];
throttle_430 = [0;0.0500000000000000;0.100000000000000;0.150000000000000;0.200000000000000;0.250000000000000;0.300000000000000;0.350000000000000;0.400000000000000;0.450000000000000;0.500000000000000;0.550000000000000;0.600000000000000;0.650000000000000;0.700000000000000;0.750000000000000;0.800000000000000;0.850000000000000;0.900000000000000;0.950000000000000;1];

y = interp1(  wrpm_430, throttle_430, wrpm, 'linear')*1000;

== matlab function controller_sim/427wrpm2throttle8 ==
  data: u input; y output
function y = fcn(u)
wrpm = u;
wrpm_430 = [3.50000000000000;4.10000000000000;4.70000000000000;5.30000000000000;5.80000000000000;6.30000000000000;6.80000000000000;7.10000000000000;7.50000000000000;7.80000000000000;8.20000000000000;8.40000000000000;8.70000000000000;8.80000000000000;9;9.10000000000000;9.30000000000000;9.40000000000000;9.50000000000000;9.60000000000000;9.70000000000000];
throttle_430 = [0;0.0500000000000000;0.100000000000000;0.150000000000000;0.200000000000000;0.250000000000000;0.300000000000000;0.350000000000000;0.400000000000000;0.450000000000000;0.500000000000000;0.550000000000000;0.600000000000000;0.650000000000000;0.700000000000000;0.750000000000000;0.800000000000000;0.850000000000000;0.900000000000000;0.950000000000000;1];

y = interp1(  wrpm_430, throttle_430, wrpm, 'linear')*1000;

== matlab function controller_sim/429throttle2wrpm1 ==
  data: u input; y output
function y = fcn(u)
throttle = u/1000.0;
wrpm_430 = [3.60000000000000;4.20000000000000;4.80000000000000;5.30000000000000;5.90000000000000;6.40000000000000;6.80000000000000;7.20000000000000;7.50000000000000;7.80000000000000;8.10000000000000;8.40000000000000;8.70000000000000;8.90000000000000;9;9.20000000000000;9.30000000000000;9.40000000000000;9.50000000000000;9.60000000000000;9.70000000000000];
throttle_430 = [0;0.0500000000000000;0.100000000000000;0.150000000000000;0.200000000000000;0.250000000000000;0.300000000000000;0.350000000000000;0.400000000000000;0.450000000000000;0.500000000000000;0.550000000000000;0.600000000000000;0.650000000000000;0.700000000000000;0.750000000000000;0.800000000000000;0.850000000000000;0.900000000000000;0.950000000000000;1];
y = interp1(throttle_430, wrpm_430, throttle, 'linear');

== matlab function controller_sim/427wrpm2throttle5 ==
  data: u input; y output
function y = fcn(u)
wrpm = u;
wrpm_430 = [3.50000000000000;4.10000000000000;4.70000000000000;5.30000000000000;5.80000000000000;6.30000000000000;6.80000000000000;7.10000000000000;7.50000000000000;7.80000000000000;8.20000000000000;8.40000000000000;8.70000000000000;8.80000000000000;9;9.10000000000000;9.30000000000000;9.40000000000000;9.50000000000000;9.60000000000000;9.70000000000000];
throttle_430 = [0;0.0500000000000000;0.100000000000000;0.150000000000000;0.200000000000000;0.250000000000000;0.300000000000000;0.350000000000000;0.400000000000000;0.450000000000000;0.500000000000000;0.550000000000000;0.600000000000000;0.650000000000000;0.700000000000000;0.750000000000000;0.800000000000000;0.850000000000000;0.900000000000000;0.950000000000000;1];

y = interp1(  wrpm_430, throttle_430, wrpm, 'linear')*1000;
